simulink model "doubleIt_01"  (R2020b)
settings: Solver=FixedStepAuto  StartTime=0.0  StopTime=0.5  FixedStep=1e-4  RelTol=1e-3
settings Model: Creator=Kasper Laustsen  LastModifiedBy=Kasper Laustsen

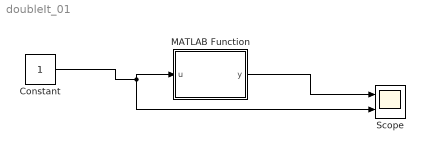
== system doubleIt_01 ==
  Constant : Constant
  MATLAB Function : MATLAB Function  TreatAsAtomicUnit=on
  Scope : Scope  NumInputPorts=2
  wires:
  Constant/1 -> Scope/2, MATLAB Function/1(u)
  MATLAB Function/1(y) -> Scope/1

== matlab function doubleIt_01/MATLAB Function ==
  data: u input; y output
function y = callingDoubleIt(u)
coder.updateBuildInfo('addSourceFiles','doubleIt.c');
coder.cinclude('doubleIt.h');

y = 0.0;


y = coder.ceval('doubleIt',u);
